simulink model "power_transfohyst"  (Simulink 6.0)
settings: Solver=ode23tb  SolverMode=SingleTasking  StartTime=0.0  StopTime=0.14  FixedStep=50e-6  RelTol=1e-4
undefined symbols (not defined in the file or in its folder): Current, DiscIntNeverNeededParam, HT, LowerFlux, sfun_InitialFlux, Tolerances, UpperFlux
libraries: powerlib x9, simulink x1, powerlib_models x1
settings Model: Creator=patrice  LastModifiedBy=batserve  ExtModeTrigMode=oneshot  ExtModeArmWhenConnect=off  ExtModeAutoUpdateStatusClock=off
settings DataIOCC: LimitDataPoints=off  SignalLoggingName=sigsOut
settings OptimizationCC: BlockReduction=off  BooleanDataType=off
settings DebuggingCC: CheckExecutionContextPreStartOutputMsg=on  CheckExecutionContextRuntimeOutputMsg=on  SolverPrmCheckMsg=none
settings HardwareCC: TargetUnknown=on
settings RTWCC: TemplateMakefile=grt_unix.tmf

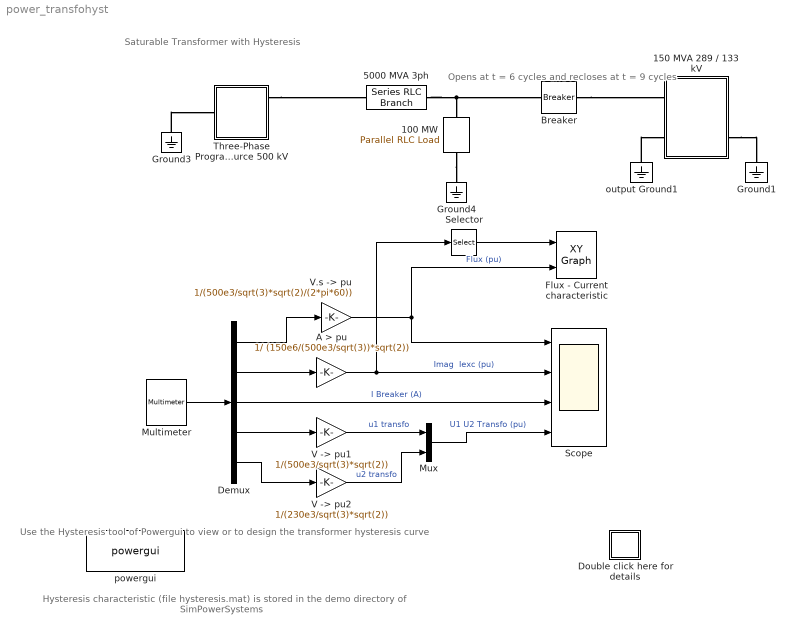
== system power_transfohyst ==
  note: Saturable Transformer with Hysteresis
  note: Hysteresis characteristic (file hysteresis.mat)
      | is stored in the demo directory of
      | SimPowerSystems
  note: Opens at t = 6 cycles
      | and recloses at  t = 9 cycles
  note: Use the Hysteresis tool of Powergui to view
      | or to design the transformer hysteresis curve
  100 MW : powerlib/Elements/Parallel RLC Load  Orientation=down  PhysicalDomain=powersysdomain  SubClassName=unknown  LeftPortType=p1  RightPortType=p1  LConnTagsString=a  RConnTagsString=__new0  NominalVoltage=500e3/sqrt(3)  NominalFrequency=60  ActivePower=100e6  InductivePower=0  CapacitivePower=0  Measurements=None
      settings: AttributesFormatString=\n
  150 MVA 289 / 133 kV : Subsystem  LoadFcn=|  mask(Saturable Transformer){NominalPower=[ 150e6 60 ], Winding1=[ 500e3/sqrt(3) 0.002 0.08 ], Winding2=[ 230e3/sqrt(3) 0.002 0.08], ThreeWindings=off, Winding3=[ 230e3/sqrt(3) 0.002 0.08], Saturation=[0 0;  0.0 0.85; 0.015 1.2;  0.03 1.35; 0.06 1.5; 0.09 1.56; 0.12 1.572], CoreLoss=[200 0], Hysteresis=on, DataFile='hysteresis', Measurements=All measurements (V I Flux), InitialFlux=-51.8986800285954, TransfoNumber=1}
      | try                                  
      | set_param(gcb,'Linkstatus','restore')
      | end
      mask prompts: NominalPower "Nominal power and frequency [Pn(VA) fn(Hz)]:"; Winding1 "Winding 1 parameters [V1(Vrms) R1(pu) L1(pu)]:"; Winding2 "Winding 2 parameters [V2(Vrms) R2(pu) L2(pu)]:"; ThreeWindings "Three windings transformer"; Winding3 "Winding 3 parameters [V3(Vrms) R3(pu) L3(pu)]:"; Saturation "Saturation characteristic [i1(pu) phi1(pu); i2 phi2; ...]:"; CoreLoss "Core loss resistance and initial flux [Rm(pu) phi0(pu)] or [Rm(pu)] only:"; Hysteresis "Simulate hysteresis"; DataFile "Hysteresis Data Mat file"; InitialFlux "Initial Flux (internal use)"; TransfoNumber "Device number (internal use)"
      mask help: Three windings linear transformer.
      mask init:
      | block = gcb;
      | [p1,p2,p3,p4,p5,p6,p7,p8,mot,t1]=powericon('SaturableTransformerIcon',ThreeWindings);
      | %
      | powerbase = NominalPower(1);
      | wbase = 2*pi*NominalPower(2);
      | voltbase = Winding1(1);
      | BaseCurrent = (powerbase/voltbase)*sqrt(2);
      | BaseFlux = (voltbase/wbase)*sqrt(2);
      | Saturation = [-Saturation(size(Saturation,1):-1:2,:) ; Saturation(2:size(Saturation,1),:)];
      | SaturationCurrent = [Saturation(:,1)*BaseCurrent]';
      | SaturationFlux = [Saturation(:,2)*BaseFlux]'; 
      | if length(CoreLoss)==2
      |     InitialFlux = CoreLoss(2)*BaseFlux;
      | end
      | if Hysteresis
      |     InitialSlope = 1;
      | 	[sfun_InitialFlux,Tolerances,HT,UpperFlux,LowerFlux,Current] = powericon('inithysteresis',DataFile,BaseFlux,BaseCurrent,InitialFlux);
      | 	if HT.UnitsPopup == 2
      | 		% The hysteresis characteristic is in S.I.
      | 		% consequentely we do not need to convert the in/out signals
      | 		% of the sfunction
      | 		BaseCurrent = 1;
      | 		BaseFlux = 1;
      | 	end	
      | end
      | %
      | Ts = powericon('SaturableTransformerInit',block);
      | powericon('SaturableTransformerCback',block);
      | powericon('psbloadfunction',block,'gotogotofrom','Initialize');
      settings: AttributesFormatString=\n  CopyFcn=powericon('psbloadfunction',gcb,'gotogotofrom','UpdateGotoTag');
      mask Help: web(psbhelp)
      mask StyleString: edit,edit,edit,checkbox,edit,edit,edit,checkbox,edit,popup(None|Winding voltages|Winding currents|Flux and excitation current ( Imag + IRm )|Flux and magnetization current ( Imag )|All measurements (V I Flux)),edit,edit
      mask CallbackString: |||powericon('SaturableTransformerCback',gcb);||||powericon('SaturableTransformerCback',gcb);||||
      mask Display:
      | plot(-85,-100,85,100,p1,p2,p3,p4,p5,p6,p7,p8);
      | text(-85,0, '1');
      | text(70,t1, '2');
      | text(70,-50, mot);
  5000 MVA 3ph : powerlib/Elements/Series RLC Branch  PhysicalDomain=powersysdomain  SubClassName=unknown  LeftPortType=p1  RightPortType=p1  LConnTagsString=__new0  RConnTagsString=__new0  Resistance=500e3^2/5000e6/10  Inductance=500e3^2/5000e6/(2*pi*60)  Capacitance=inf  Measurements=Branch current
  A > pu : Gain  Gain=1/ (150e6/(500e3/sqrt(3))*sqrt(2))  SaturateOnIntegerOverflow=on
  Breaker : powerlib/Elements/Breaker  BreakerResistance=0.01  InitialState=1  SnubberResistance=1e7  SnubberCapacitance=inf  SwitchingTimes="[ 6/60  9/60]"  External=off  Measurements=None
      settings: AttributesFormatString=\n
  Demux : Demux  Outputs="[1 2 1  1  1]"
  Double click here for details : Subsystem
      mask Display: disp('?')
  Flux - Current characteristic : simulink/Sinks/XY Graph  xmin=-0.05  xmax=0.05  ymin=-1.5  ymax=1.5  st=-1
  Ground1 : powerlib/Elements/Ground  Orientation=down  PhysicalDomain=powersysdomain  SubClassName=unknown  LeftPortType=p1  RightPortType=p1  LConnTagsString=a
  Ground3 : powerlib/Elements/Ground  Orientation=down  PhysicalDomain=powersysdomain  SubClassName=unknown  LeftPortType=p1  RightPortType=p1  LConnTagsString=a
  Ground4 : powerlib/Elements/Ground  Orientation=down  PhysicalDomain=powersysdomain  SubClassName=unknown  LeftPortType=p1  RightPortType=p1  LConnTagsString=a
  Multimeter : powerlib/Measurements/Multimeter  Tag=PoWeRsYsTeMmEaSuReMeNt  PhasorSimulation=off  OutputType=Magnitude  sel=[8 7 6 4 1 2]  L=8  Gain=[1 1 1 1 1 1]  yselected={'Flux: 150 MVA 289 // 133 kV','Imag: 150 MVA 289 // 133 kV','Iexc: 150 MVA 289 // 133 kV','Iw1: 150 MVA 289 // 133 kV','Uw1: 150 MVA 289 // 133 kV','Uw2: 150 MVA 289 // 133 kV'};  PSBOutputType=1  PSBequivalent=1  AxesSetting=[0,0.1,-100,100]  Display=0  SavedBlockNames=-11
      settings: AttributesFormatString=\n
  Mux : Mux  Inputs=2
  Scope : Scope  NumInputPorts=4
      settings: DeleteFcn=simscope BlockIsBeingDestroyed  PostSaveFcn=simscope Save  TimeRange=0.14  YMin=-2~-0.0153499~-200~-2  YMax=2~0.0178204~600~2  DataFormat=Array
  Selector : Selector  InputPortWidth=2
  Three-Phase Programmable Voltage Source 500 kV : Subsystem  AncestorBlock=|  mask(Three-Phase Programmable Voltage Source){PositiveSequence=[0.8*500e3  90  60], VariationEntity=Amplitude, VariationType=Step, VariationStep=0.375, VariationRate=10, VariationMagnitude=0.3, VariationFrequency=2, VariationTiming=[0.05 1], VariationPhaseA=off, Amplitudes=[1 0.8 1.2 1.0], TimeValues=[0 0.1 0.15 0.2], HarmonicGeneration=off, HarmonicA=[3 0.2 -25 0], HarmonicB=[2 0.15 35 2], Timing=[0.05  3]}
      | powerlib/Electrical
      | Sources/Three-Phase
      | Programmable
      | Voltage Source
      mask prompts: PositiveSequence "Positive-sequence: [ Amplitude(Vrms Ph-Ph)  Phase(deg.)   Freq. (Hz) ]"; VariationEntity "Time variation of:"; VariationType "Type of variation:"; VariationStep "Step magnitude (pu, Hz or deg.):"; VariationRate "Rate of change (pu/s, Hz/s or deg/s):"; VariationMagnitude "Amplitude of the modulation (pu, Hz or deg.):"; VariationFrequency "Frequency of the modulation(Hz):"; VariationTiming "Variation timing (s) : [ Start   End ]"; VariationPhaseA "Variation on phase A only"; Amplitudes "Amplitude values (pu):"; TimeValues "Time values:"; HarmonicGeneration "Fundamental and/or Harmonic generation:"; HarmonicA "A:  [ Order(n)   Amplitude(pu) Phase(degrees)  Seq(0, 1 or 2) ]"; HarmonicB "B:  [ Order(n)   Amplitude(pu) Phase(degrees)  Seq(0, 1 or 2) ]"; Timing "Timing (s) : [ Start   End ]"
      mask help:
      | This block implements a three-phase zero-impedance voltage source. The common node (neutral) of the three sources is accessible via input 1 (N) of the block. Time variation for the amplitude, phase and frequency of the fundamental can be pre-programmed. In addition, two harmonics can be surimposed on the fundamental.
      |
      | Note: For  "Phasor simulation" , frequency variation and harmonic injection are not allowed.  Specify  Order =1 and Seq=1,2 or 0 to inject additional fundamendal components A and B in  any sequence.
      mask init:
      | block=gcb;
      | % Extra variable:
      | SinglePhase=0;
      | 
      | % Conversion of pos. seq.amplitude from Ph-Ph rms voltage to Phase-gnd peak
      | MagnitudeVps = PositiveSequence(1)*sqrt(2/3);
      | PhaseVps = PositiveSequence(2);
      | FreqVps = PositiveSequence(3);
      | 
      | % Conversion of harmonic amplitudes from pu to Phase-gnd peak volt
      | HarmonicA(2) = HarmonicA(2)*MagnitudeVps;
      | HarmonicB(2) = HarmonicB(2)*MagnitudeVps;
      | 
      | % Conversion of amplitude variation from pu to Ph-G peak volt
      | if VariationEntity==2
      | 	VariationStep = VariationStep*MagnitudeVps;
      | 	VariationRate = VariationRate*MagnitudeVps;
      | 	VariationMagnitude  = VariationMagnitude*MagnitudeVps;
      | 	Amplitudes = Amplitudes*MagnitudeVps;
      | end
      | 
      | % extract other parameters
      | Ton_Variation = VariationTiming(1);
      | Toff_Variation = VariationTiming(2);
      | %
      | n_HarmoA = HarmonicA(1);
      | Mag_HarmoA = HarmonicA(2);
      | Phase_HarmoA = HarmonicA(3);
      | Seq_HarmoA = HarmonicA(4);
      | if n_HarmoA==0
      |     Phase_HarmoA = 90;
      |     Seq_HarmoA = 0;
      | end
      | %
      | n_HarmoB = HarmonicB(1);
      | Mag_HarmoB = HarmonicB(2);
      | Phase_HarmoB = HarmonicB(3);
      | Seq_HarmoB = HarmonicB(4);
      | if n_HarmoB==0
      |     Phase_HarmoB = 90;
      |     Seq_HarmoB = 0;
      | end
      | %
      | Ton_Harmo = Timing(1);
      | Toff_Harmo = Timing(2);
      | %
      | if TimeValues(1)~=0,
      |     TimeValues=[0 TimeValues];
      |     Amplitudes=[0 Amplitudes];
      | end
      | %
      | n = length(TimeValues); 
      | vec_dt = [TimeValues,0] - [0,TimeValues];
      | vec_dt = vec_dt(2:n);
      | %
      | powericon('psbloadfunction',block,'goto','Initialize');
      | Ts = powericon('ThreePhaseProgSourceInit',block);
      settings: CopyFcn=powericon('psbloadfunction',gcb,'goto','UpdateGotoTag');
      mask Help: web(psbhelp)
      mask StyleString: edit,popup(None|Amplitude|Phase|Frequency),popup(Step|Ramp|Modulation|Table of time-amplitude pairs),edit,edit,edit,edit,edit,checkbox,edit,edit,checkbox,edit,edit,edit
      mask CallbackString: |powericon('ProgrammableVoltageSourceCback',gcb);|powericon('ProgrammableVoltageSourceCback',gcb);|||||||||powericon('ProgrammableVoltageSourceCback',gcb);|||
      mask Display: plot(-80,-50,80,50,[0,9,18,24,29,30,29,24,18,9,0,-9,-18,-24,-29,-30,-29,-24,-18,-9,0],[30,29,24,18,9,0,-9,-18,-24,-29,-30,-29,-24,-18,-9,0,9,18,24,29,30],[-50 -30],[0 0],[50,30],[0 0],[45 35 40 40 40],[15 15 15 20 10],[1 2 3 4 5 6 7 8 9 10 11 12 13 14 15 16 17 18 19 20 21].*1.5-15,[0,9,18,24,29,30,29,24,18,9,0,-9,-18,-24,-29,-30,-29,-24,-18,-9,0]./2.4)
  "V -> pu1" : Gain  Gain=1/(500e3/sqrt(3)*sqrt(2))  SaturateOnIntegerOverflow=on
  "V -> pu2" : Gain  Gain=1/(230e3/sqrt(3)*sqrt(2))  SaturateOnIntegerOverflow=on
  "V.s -> pu" : Gain  Gain=1/(500e3/sqrt(3)*sqrt(2)/(2*pi*60))  SaturateOnIntegerOverflow=on
  output Ground1 : powerlib/Elements/Ground  Orientation=down  PhysicalDomain=powersysdomain  SubClassName=unknown  LeftPortType=p1  RightPortType=p1  LConnTagsString=a
  powergui : powerlib/powergui  Priority=2  Frange=[0:2:500]  Ylog=off  Xlog=on  save=off  variable=ZData  ZoomFFT=on  StartTime=0.0  cycles=1  DisplayStyle=off  fundamental=60  FreqAxis=off  MaxFrequency=1000  frequencyindice=1  frequencyindicesteady=1  RmsSteady=1  display=off  Ts=25e-6  methode=off  frequency=60  echomessages=off
  wires:
  Demux/1 -> "V.s -> pu"/1
  "V.s -> pu"/1 -> Flux - Current characteristic/2, Scope/1  "Flux (pu)"
  "V -> pu1"/1 -> Mux/1  "u1 transfo"
  "V -> pu2"/1 -> Mux/2  "u2 transfo"
  Mux/1 -> Scope/4  "U1 U2 Transfo (pu)"
  A > pu/1 -> Scope/2, Selector/1  "Imag  Iexc (pu)"
  Demux/2 -> A > pu/1
  Demux/3 -> Scope/3  "I Breaker (A)"
  Demux/4 -> "V -> pu1"/1
  Demux/5 -> "V -> pu2"/1
  Multimeter/1 -> Demux/1
  Selector/1 -> Flux - Current characteristic/1
  connections:
  5000 MVA 3ph/RConn1 -- Breaker/LConn1 -- 100 MW/LConn1
  150 MVA 289 / 133 kV/RConn2 -- Ground1/LConn1
  Breaker/RConn1 -- 150 MVA 289 / 133 kV/LConn1
  Three-Phase Programmable Voltage Source 500 kV/RConn1 -- 5000 MVA 3ph/LConn1
  100 MW/RConn1 -- Ground4/LConn1
  output Ground1/LConn1 -- 150 MVA 289 / 133 kV/LConn2
  Ground3/LConn1 -- Three-Phase Programmable Voltage Source 500 kV/LConn1

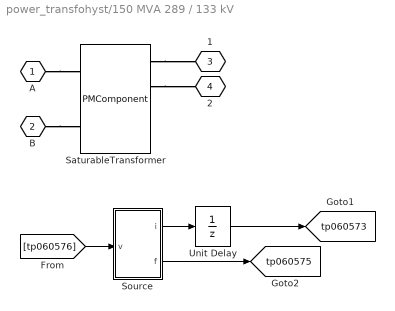
== system power_transfohyst/150 MVA 289 / 133 kV ==
  SaturableTransformer : PMComponent  PhysicalDomain=powersysdomain  LeftPortType=p1  RightPortType=p1  LConnTagsString=A|B  RConnTagsString=1|2|3|4
      mask Type: InnerPowersysBlock
  Source : Subsystem  AncestorBlock=powerlib_models/Discrete/hysteresis_transformer  mask{SaturationFlux=SaturationFlux, SaturationCurrent=SaturationCurrent, InitialFlux=InitialFlux, FluxBase=BaseFlux, CurrentBase=BaseCurrent, Tolerances=Tolerances, HT=HT, UpperFlux=UpperFlux, LowerFlux=LowerFlux, Current=Current, InitialSlope=InitialSlope, TransfoNumber=TransfoNumber, Ts=Ts, sfun_InitialFlux=sfun_InitialFlux}
      mask prompts: InitialFlux "Initial Flux"; TransfoNumber "Transfo Number"
  Unit Delay : UnitDelay  SampleTime=Ts
  A : PMIOPort  Port=1  Side=Left
  B : PMIOPort  Port=2  Side=Left
  1 : PMIOPort  Orientation=left  Port=3  Side=Right
  2 : PMIOPort  Orientation=left  Port=4  Side=Right
  tag scope: tp060573=global, tp060575=global
  wires:
  Source/2(f) -> [tp060575]
  Source/1(i) -> Unit Delay/1
  [tp060576] -> Source/1(v)
  Unit Delay/1 -> [tp060573]
  connections:
  SaturableTransformer/RConn2 -- 2/RConn1
  SaturableTransformer/RConn1 -- 1/RConn1
  A/RConn1 -- SaturableTransformer/LConn1
  B/RConn1 -- SaturableTransformer/LConn2

== system power_transfohyst/Double click here for details ==
  note: S. Casoria (Hydro-Quebec) and P. Brunelle (TransEnergie)
  note: Demonstration
  note: Circuit Description
  note: This demonstration illustrates simulation of hystersis in a saturable transformer
  note: One phase of a three-phase transformer  is connected on a 500 kV, 5000 MVA network. The transformer is rated 500 kV/230 kV, 450 MVA (150 MVA per phase).
      | The flux-current saturation characteristic of the transformer is modelled with the hysteresis or with a simple  piecewise nonlinear characteristic.
      |
      | A Thrre-Phase Programmable Voltagge Source is used to vary the internal voltage of the equivalent 500 kV network.
      | During the first 3 cycles source voltage is programmed at 0.8 pu. Then, at t = 3 cycles (0.05 s) voltage is increased  by 37.5% (up to 1.10 pu).
      | In order to illustrate remanent flux and inrush current at transformer energization, the circuit breaker which is initially closed
      | is first opened at t = 6 cycles (0.1 s),  then it is reclosed at t = 9 cycles (0.15 s).
      |
      | The Initial flux phi0 in the transformer is set at zero and source phase angle is adjusted at 90 degrees so that flux remains symetrical around zero
      | when simulation is started.
      |
      | A Multimeter block and a Scope block are used to monitor waveforms of flux, magnetization current (not including the eddy currrents
      | which are modelled by the Rm resistance), excitation current (including eddy current modeled by Rm) , voltages and current flowing into primary winding.
      | A X-Y Graph block is used to monitor the transformer operating point moving on the flux-current characteristic.
  note: Open the transformer menu and select the 'Simulate hysteresis' check box.
      | Using the 'Hysteresis design' tool of the Powergui, load the hysteresis characteristic (load file 'hysteresis.mat').
      | Notice that flux and excitation current are displayed in pu. Using the 'Parameter units' popu menu, you can convert the pu units to SI units.
      | The saturation characteristics consists of two regions:
      |      1) The main hysteresis loop: In this region there are 2 different flux values for a single current value.
      |      2) The saturated region defined by a simple line segment starting from the maximum point (Is,Fs) of the main loop.
      | The hysteresis loop is defined by the following 3 points marked by red crosses on the main loop:
      |     [I=0; Remanent flux (Fr = 0.85pu)] , [Coercive Current(Ic = 0.004 pu) ; F = 0] , [Saturation current (Is = 0.015 pu); Saturation flux (Fs = 1.2 pu)]
      |     plus the slope dF/dI at coercive current (F = 0).
      | Using the 'Zoom around hysteresis' checkbox and 'Display' button you can view the whole charactersistic or zoom on the hysteresis.
      |
      | Start the simulation and observe the following phenomena on the two scope blocks:
  note: Voltage and flux peak values are at 0.8 pu. Notice typical square wave of magnetization current.
      | As no remanent flux was specified, magnetization current and flux are symetrical. Flux travels on inner loops (inside the main loop).
  note: Voltage is 1.1 pu. Flux now reaches approximately +1.1pu. A slight flux asymetry is produced at  voltage change.
      | and the flux which varies between +1.14 pu and -1.05 pu now travels on the main loop.
      | Current pulses appear on the magnetization current (yellow  trace, Imag), indicating begining of saturation.
  note: At first zero crossing after the breaker opening order, the current is interrupted, and a flux of 0.84 pu stays trapped in the transformer core.
  note: The breaker is reclosed at t = 9 cycles, at a zero crossing of source voltage, producing an additional flux offset of approximatlely 1 pu.
      | The peak flux now reaches 1.85 pu, driving the transformer into the saturated region. Peak excitation current now reaches 0.81 pu.
  note: 1) Simulation of saturation with hysteresis
  note: 2) Simulation of saturation with a piecewise nonlinear characteristic
  note: Open the transformer menu and deselect 'Simulate hysteresis'. The saturation will now be simulated by a piecewise nonlinear single-valued characteristic
      | defined by 7 points. Current/Flux pairs (in pu) are: [0 0;  0.0 0.85; 0.015 1.2;  0.03 1.35; 0.06 1.5; 0.09 1.56; 0.12 1.572].
      | The saturated region is the same, but the hysteresis loop is not simulated. Note that  this single valued characteristics still allows specifation
      | of a remanent flux  ( keep phi0=0 flux as with hysteresis saturation model).
      | Start simulation and compare waveforms.
  note: From 0 to 0.05 sec:
  note: From 0.05 to 0.1 sec:
  note: From 0.1 to 0.15 sec:
  note: From 0.15 to 0.2 sec :

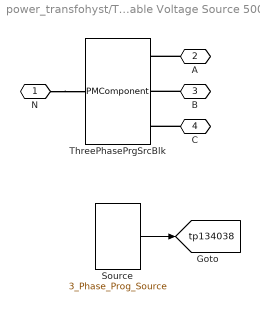
== system power_transfohyst/Three-Phase Programmable Voltage Source 500 kV ==
  Source : powerlib_models/Discrete/3_Phase_Prog_Source  SimViewingDevice=off  DataTypeOverride=UseLocalSettings  MinMaxOverflowLogging=UseLocalSettings
      settings: Permissions=ReadWrite  RTWFcnNameOpts=Auto  RTWFileNameOpts=Auto
  ThreePhasePrgSrcBlk : PMComponent  PhysicalDomain=powersysdomain  LeftPortType=p1  RightPortType=p1  LConnTagsString=N  RConnTagsString=A|B|C
      mask Type: InnerPowersysBlock
  N : PMIOPort  Port=1  Side=Left
  A : PMIOPort  Orientation=left  Port=2  Side=Right
  B : PMIOPort  Orientation=left  Port=3  Side=Right
  C : PMIOPort  Orientation=left  Port=4  Side=Right
  tag scope: tp134038=global
  wires:
  Source/1 -> [tp134038]
  connections:
  C/RConn1 -- ThreePhasePrgSrcBlk/RConn3
  B/RConn1 -- ThreePhasePrgSrcBlk/RConn2
  N/RConn1 -- ThreePhasePrgSrcBlk/LConn1
  A/RConn1 -- ThreePhasePrgSrcBlk/RConn1

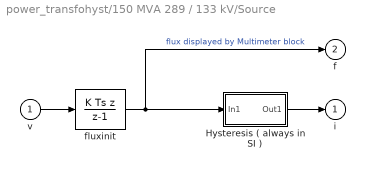
== system power_transfohyst/150 MVA 289 / 133 kV/Source ==
  v : Inport  Port=1  LatchInput=off
  Hysteresis ( always in SI ) : Subsystem
  fluxinit : DiscreteIntegrator  IntegratorMethod=Integration: Backward Euler  InitialCondition=InitialFlux  SampleTime=Ts  ICPrevOutput=DiscIntNeverNeededParam  ICPrevScaledInput=DiscIntNeverNeededParam
  i : Outport  InitialOutput=0
  f : Outport  Port=2  InitialOutput=0
  wires:
  Hysteresis ( always in SI )/1(Out1) -> i/1
  fluxinit/1 -> f/1, Hysteresis ( always in SI )/1(In1)  "flux displayed by Multimeter block"
  v/1 -> fluxinit/1

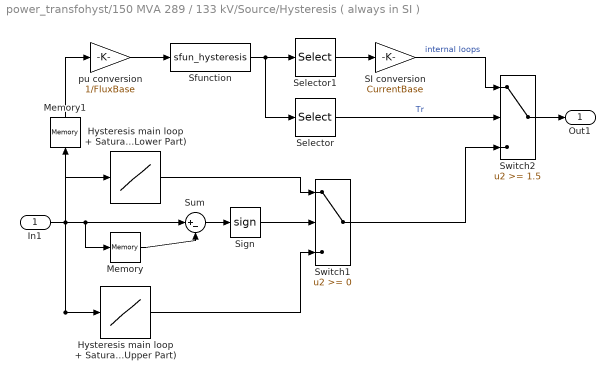
== system power_transfohyst/150 MVA 289 / 133 kV/Source/Hysteresis ( always in SI ) ==
  In1 : Inport  Port=1  LatchInput=off
  Hysteresis main loop + Saturation (Lower Part) : Lookup  DialogController=Simulink.DDGSource  InputValues=LowerFlux  OutputValues=Current  SaturateOnIntegerOverflow=on
  Hysteresis main loop + Saturation. (Upper Part) : Lookup  DialogController=Simulink.DDGSource  InputValues=UpperFlux  OutputValues=Current  SaturateOnIntegerOverflow=on
  Memory : Memory
  Memory1 : Memory  Orientation=up
  SI conversion : Gain  Gain=CurrentBase  SaturateOnIntegerOverflow=on
  Selector : Selector  Elements=2  InputPortWidth=2
  Selector1 : Selector  InputPortWidth=2
  Sfunction : S-Function  FunctionName=sfun_hysteresis  Parameters=sfun_InitialFlux,HT,TransfoNumber,Ts,Tolerances,InitialSlope
  Sign : Signum
  Sum : Sum  Inputs=|+-  SaturateOnIntegerOverflow=on  InputSameDT=on
  Switch1 : Switch  InputSameDT=on
  Switch2 : Switch  Threshold=1.5  InputSameDT=on
  pu conversion : Gain  Gain=1/FluxBase  SaturateOnIntegerOverflow=on
  Out1 : Outport
  wires:
  Sum/1 -> Sign/1
  SI conversion/1 -> Switch2/1  "internal loops"
  Selector1/1 -> SI conversion/1
  Selector/1 -> Switch2/2  "Tr"
  Switch1/1 -> Switch2/3
  Switch2/1 -> Out1/1
  Sfunction/1 -> Selector1/1, Selector/1
  pu conversion/1 -> Sfunction/1
  Sign/1 -> Switch1/2
  Memory/1 -> Sum/2
  Hysteresis main loop + Saturation. (Upper Part)/1 -> Switch1/3
  In1/1 -> Hysteresis main loop + Saturation. (Upper Part)/1, Memory1/1, Sum/1, Memory/1, Hysteresis main loop + Saturation (Lower Part)/1
  Hysteresis main loop + Saturation (Lower Part)/1 -> Switch1/1
  Memory1/1 -> pu conversion/1
